simulink model "Simulink"  (R2022b)
settings: Solver=VariableStepAuto  StartTime=0.0  StopTime=5  RelTol=1e-3
undefined symbols (not defined in the file): g, l, M, m
settings Model: Creator=lenovo  LastModifiedBy=lenovo

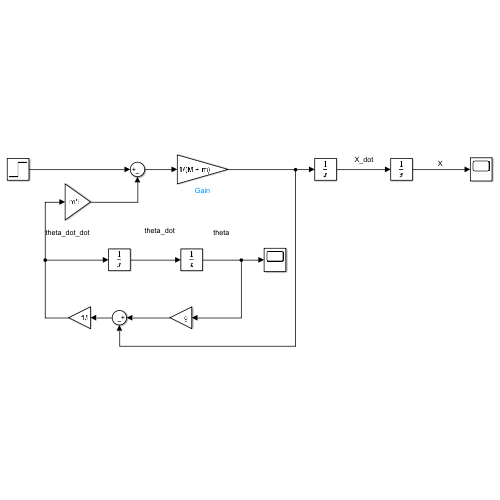
[thumbnail: Simulink's stored preview of the top-level diagram]
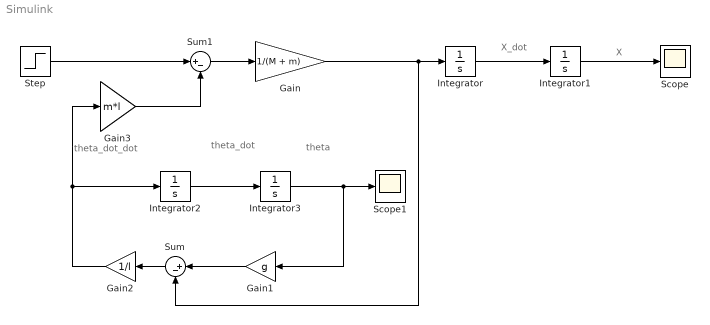
== system Simulink ==
  note: theta_dot_dot
  note: X
  note: X_dot
  note: theta_dot
  note: theta
  Gain : Gain  Gain=1/(M + m)
  Gain1 : Gain  Gain=g
  Gain2 : Gain  Gain=1/l
  Gain3 : Gain  Gain=m*l
  Integrator{,1..3} (4 alike) : Integrator
  Scope : Scope
  Scope1 : Scope
  Step : Step  Time=0  After=3  SampleTime=0
  Sum : Sum  Inputs=|+-
  Sum1 : Sum  Inputs=|+-
  wires:
  Integrator/1 -> Integrator1/1
  Integrator1/1 -> Scope/1
  Integrator2/1 -> Integrator3/1
  Gain/1 -> Sum/2, Integrator/1
  Integrator3/1 -> Gain1/1, Scope1/1
  Gain1/1 -> Sum/1
  Sum/1 -> Gain2/1
  Gain2/1 -> Gain3/1, Integrator2/1
  Gain3/1 -> Sum1/2
  Step/1 -> Sum1/1
  Sum1/1 -> Gain/1
